simulink model "HybridFEMModel"  (Simulink 7.0)
settings: Solver=FixedStepDiscrete  SolverMode=SingleTasking  StartTime=0.0  StopTime=RunningTime  FixedStep=SampleRate  RelTol=1e-3
values from neighbouring files (symbols this model uses):
  SampleRate = Integrator.Timestep    [HybridFEMSetup_1.m]
undefined symbols (not defined in the file or in its folder): Elements
libraries: simulink x2
(part 1 of 2)
settings Model: Creator=Tommy  LastModifiedBy=Tommy

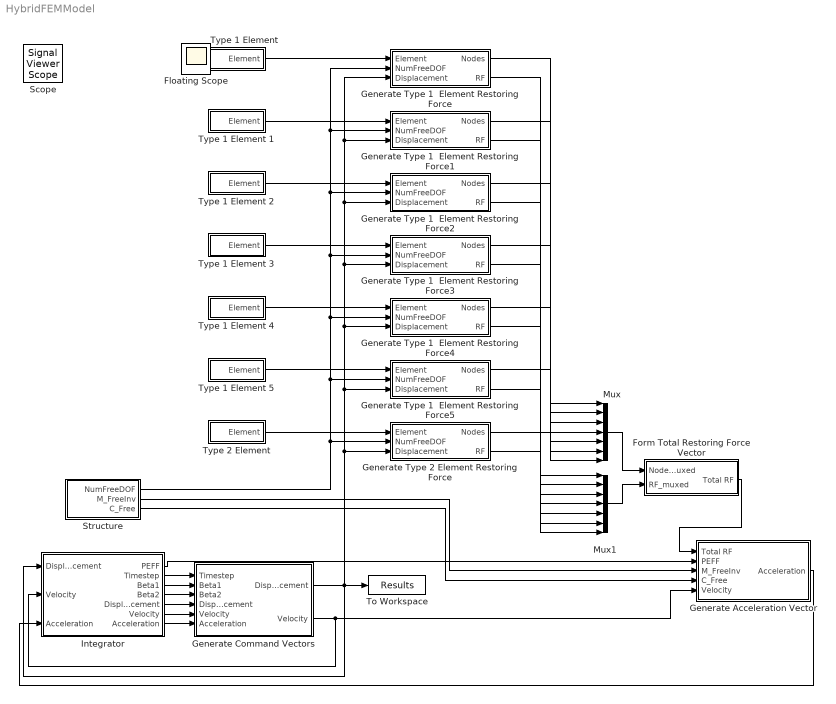
== system HybridFEMModel ==
  Form Total Restoring Force Vector : Subsystem
      mask Type: Form Restoring Force Vector
      mask Description:
      | Takes the restoring force vectors from each Element and combines them to form a total restoring force vector.
      | 
      | Connect the "Nodes_muxed" signal to the output of a Mux block which takes in all the Element "Nodes" outputs in order of ID.
      | 
      | Connect the "RF_muxed" signal to the output of a Mux block which takes in all the Element "RF" outputs in order of ID.
  Generate Acceleration Vector : Subsystem
      mask Type: Generate Acceleration Vector
      mask Description:
      | Takes the total restoring force vector and Integration parameters and generates the next step acceleration vector.
      | 
      | Connect the "Total RF" input to the output of the "Form Total Restoring Force Vector" block.
      | 
      | Connect the "PEFF", "M_Free_Inv" (MassMatrixFreeInv) and "C_Free" (DampingMatrixFree) to the "Structure" block.
      | 
      | Connect the "Velocity" input to the output of the "Generate Command Vectors" block
  Generate Command Vectors : Subsystem
      mask Type: Generate Command Vectors
      mask Description:
      | Generates the Displacement and Velocity vectors using the CR Algorithm.
      | 
      | Connect all inputs to the outputs of the "Integrator" block.
  Generate Type 1  Element Restoring Force : Subsystem
      mask Type: Generate Type 1 Element Restoring Force
      mask Description:
      | Generates the Restoring Force vector for a Type 1 Element
      | 
      | Connect the "Element" input to a "Type 1 Element" block.
      | 
      | Connect the "NumFreeDOF" input to the output of a "Structure" block.
      | 
      | Connect the "Displacement" input to the output of the "Generate Command Vectors" block.
  Generate Type 1  Element Restoring Force1 : Subsystem
      mask Type: Generate Type 1 Element Restoring Force
      mask Description:
      | Generates the Restoring Force vector for a Type 1 Element
      | 
      | Connect the "Element" input to a "Type 1 Element" block.
      | 
      | Connect the "NumFreeDOF" input to the output of a "Structure" block.
      | 
      | Connect the "Displacement" input to the output of the "Generate Command Vectors" block.
  Generate Type 1  Element Restoring Force2 : Subsystem
      mask Type: Generate Type 1 Element Restoring Force
      mask Description:
      | Generates the Restoring Force vector for a Type 1 Element
      | 
      | Connect the "Element" input to a "Type 1 Element" block.
      | 
      | Connect the "NumFreeDOF" input to the output of a "Structure" block.
      | 
      | Connect the "Displacement" input to the output of the "Generate Command Vectors" block.
  Generate Type 1  Element Restoring Force3 : Subsystem
      mask Type: Generate Type 1 Element Restoring Force
      mask Description:
      | Generates the Restoring Force vector for a Type 1 Element
      | 
      | Connect the "Element" input to a "Type 1 Element" block.
      | 
      | Connect the "NumFreeDOF" input to the output of a "Structure" block.
      | 
      | Connect the "Displacement" input to the output of the "Generate Command Vectors" block.
  Generate Type 1  Element Restoring Force4 : Subsystem
      mask Type: Generate Type 1 Element Restoring Force
      mask Description:
      | Generates the Restoring Force vector for a Type 1 Element
      | 
      | Connect the "Element" input to a "Type 1 Element" block.
      | 
      | Connect the "NumFreeDOF" input to the output of a "Structure" block.
      | 
      | Connect the "Displacement" input to the output of the "Generate Command Vectors" block.
  Generate Type 1  Element Restoring Force5 : Subsystem
      mask Type: Generate Type 1 Element Restoring Force
      mask Description:
      | Generates the Restoring Force vector for a Type 1 Element
      | 
      | Connect the "Element" input to a "Type 1 Element" block.
      | 
      | Connect the "NumFreeDOF" input to the output of a "Structure" block.
      | 
      | Connect the "Displacement" input to the output of the "Generate Command Vectors" block.
  Generate Type 2 Element Restoring Force : Subsystem
      mask Type: Generate Type 2 Element Restoring Force
      mask Description:
      | Generates the Restoring Force vector for a Type 2 Element
      | 
      | Connect the "Element" input to a "Type 2 Element" block.
      | 
      | Connect the "NumFreeDOF" input to the output of a "Structure" block.
      | 
      | Connect the "Displacement" input to the output of the "Generate Command Vectors" block.
  Integrator : Subsystem
      mask Type: Integrator
      mask Description:
      | The Integrator structure is pulled from the MATLAB workspace after running the initialization script.
      | 
      | Connect the Displacement and Velocity inputs to the outputs of the "Generate Command Vectors" block.
      | 
      | Connect the Acceleration input to the output of the "Generate Acceleration Vector" block
  Mux : Mux  Inputs=7
  Mux1 : Mux  Inputs=7
  Structure : Subsystem
      mask Type: Structure Data Source
      mask Description: The Structure data is pulled from the MATLAB workspace after running the initialization file
  To Workspace : ToWorkspace  VariableName=Results  SampleTime=SampleRate  SaveFormat=Array
  "Type 1 Element " : Subsystem  mask(Element Type 1){id=1}
      mask prompts: id "Element ID:"
      mask help: Enter the ID for this element corresponding with the input configuration file
  Type 1 Element 1 : Subsystem  mask(Element Type 1){id=2}
      mask prompts: id "Element ID:"
      mask help: Enter the ID for this element corresponding with the input configuration file
  Type 1 Element 2 : Subsystem  mask(Element Type 1){id=3}
      mask prompts: id "Element ID:"
      mask help: Enter the ID for this element corresponding with the input configuration file
  Type 1 Element 3 : Subsystem  mask(Element Type 1){id=4}
      mask prompts: id "Element ID:"
      mask help: Enter the ID for this element corresponding with the input configuration file
  Type 1 Element 4 : Subsystem  mask(Element Type 1){id=5}
      mask prompts: id "Element ID:"
      mask help: Enter the ID for this element corresponding with the input configuration file
  Type 1 Element 5 : Subsystem  mask(Element Type 1){id=6}
      mask prompts: id "Element ID:"
      mask help: Enter the ID for this element corresponding with the input configuration file
  Type 2 Element : Subsystem  mask(Element Type 2){id=7}
      mask prompts: id "Element ID:"
      mask help: Enter the ID for this element corresponding with the input configuration file
  Floating Scope : Scope
      settings: Floating=on
  Scope : SignalViewerScope  IOType=viewer  RefreshTime=0.035000
  wires:
  "Type 1 Element "/1(Element) -> Generate Type 1  Element Restoring Force/1(Element)
  Type 1 Element 1/1(Element) -> Generate Type 1  Element Restoring Force1/1(Element)
  Type 1 Element 2/1(Element) -> Generate Type 1  Element Restoring Force2/1(Element)
  Type 1 Element 3/1(Element) -> Generate Type 1  Element Restoring Force3/1(Element)
  Type 1 Element 4/1(Element) -> Generate Type 1  Element Restoring Force4/1(Element)
  Type 1 Element 5/1(Element) -> Generate Type 1  Element Restoring Force5/1(Element)
  Type 2 Element/1(Element) -> Generate Type 2 Element Restoring Force/1(Element)
  Integrator/5(Displacement) -> Generate Command Vectors/4("Displacement ")
  Structure/1(NumFreeDOF) -> Generate Type 1  Element Restoring Force/2(NumFreeDOF), Generate Type 1  Element Restoring Force1/2(NumFreeDOF), Generate Type 1  Element Restoring Force2/2(NumFreeDOF), Generate Type 1  Element Restoring Force3/2(NumFreeDOF), Generate Type 1  Element Restoring Force4/2(NumFreeDOF), Generate Type 1  Element Restoring Force5/2(NumFreeDOF), Generate Type 2 Element Restoring Force/2(NumFreeDOF)
  Generate Command Vectors/1(Displacement) -> Generate Type 1  Element Restoring Force/3(Displacement), Generate Type 1  Element Restoring Force1/3(Displacement), Generate Type 1  Element Restoring Force2/3(Displacement), Generate Type 1  Element Restoring Force3/3(Displacement), Generate Type 1  Element Restoring Force4/3(Displacement), Generate Type 1  Element Restoring Force5/3(Displacement), Generate Type 2 Element Restoring Force/3(Displacement), Integrator/1("Displacement "), To Workspace/1
  Form Total Restoring Force Vector/1(Total RF) -> Generate Acceleration Vector/1(Total RF)
  Mux/1 -> Form Total Restoring Force Vector/1(Nodes_Muxed)
  Mux1/1 -> Form Total Restoring Force Vector/2(RF_muxed)
  Generate Type 1  Element Restoring Force/1(Nodes) -> Mux/1
  Generate Type 1  Element Restoring Force1/1(Nodes) -> Mux/2
  Generate Type 1  Element Restoring Force2/1(Nodes) -> Mux/3
  Generate Type 1  Element Restoring Force3/1(Nodes) -> Mux/4
  Generate Type 1  Element Restoring Force4/1(Nodes) -> Mux/5
  Generate Type 1  Element Restoring Force5/1(Nodes) -> Mux/6
  Generate Type 2 Element Restoring Force/1(Nodes) -> Mux/7
  Generate Type 1  Element Restoring Force/2(RF) -> Mux1/1
  Generate Type 1  Element Restoring Force1/2(RF) -> Mux1/2
  Generate Type 1  Element Restoring Force2/2(RF) -> Mux1/3
  Generate Type 1  Element Restoring Force3/2(RF) -> Mux1/4
  Generate Type 1  Element Restoring Force4/2(RF) -> Mux1/5
  Generate Type 1  Element Restoring Force5/2(RF) -> Mux1/6
  Generate Type 2 Element Restoring Force/2(RF) -> Mux1/7
  Integrator/1(PEFF) -> Generate Acceleration Vector/2(PEFF)
  Generate Command Vectors/2(Velocity) -> Integrator/2("Velocity "), Generate Acceleration Vector/5(Velocity)
  Structure/2(M_FreeInv) -> Generate Acceleration Vector/3(M_FreeInv)
  Structure/3(C_Free) -> Generate Acceleration Vector/4(C_Free)
  Generate Acceleration Vector/1(Acceleration) -> Integrator/3("Acceleration ")
  Integrator/2(Timestep) -> Generate Command Vectors/1(Timestep)
  Integrator/3(Beta1) -> Generate Command Vectors/2(Beta1)
  Integrator/4(Beta2) -> Generate Command Vectors/3(Beta2)
  Integrator/6(Velocity) -> Generate Command Vectors/5("Velocity ")
  Integrator/7(Acceleration) -> Generate Command Vectors/6(Acceleration)

== system HybridFEMModel/Form Total Restoring Force Vector ==
  Nodes_Muxed : Inport  OutDataType=sfix(16)  OutScaling=2^0
  RF_muxed : Inport  Port=2  OutDataType=sfix(16)  OutScaling=2^0
  Form Restoring Force Vector : Stateflow chart
  Total RF : Outport  OutDataType=sfix(16)  OutScaling=2^0
  wires:
  RF_muxed/1 -> Form Restoring Force Vector/2(RF_muxed)
  Form Restoring Force Vector/1(TotalRF) -> Total RF/1
  Nodes_Muxed/1 -> Form Restoring Force Vector/1(Nodes_muxed)

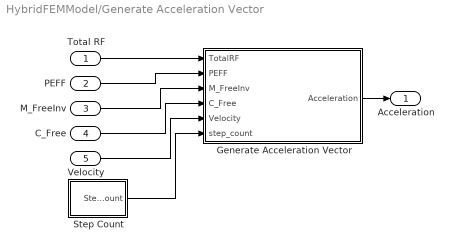
== system HybridFEMModel/Generate Acceleration Vector ==
  Total RF : Inport  OutDataType=sfix(16)  OutScaling=2^0
  PEFF : Inport  Port=2  OutDataType=sfix(16)  OutScaling=2^0
  M_FreeInv : Inport  Port=3  OutDataType=sfix(16)  OutScaling=2^0
  C_Free : Inport  Port=4  OutDataType=sfix(16)  OutScaling=2^0
  Velocity : Inport  Port=5  OutDataType=sfix(16)  OutScaling=2^0
  Generate Acceleration Vector : Stateflow chart
  Step Count : Subsystem
      mask Type: Step count
      mask Description: Generates the step count
  Acceleration : Outport  OutDataType=sfix(16)  OutScaling=2^0
  wires:
  Step Count/1(Step Count) -> Generate Acceleration Vector/6(step_count)
  Total RF/1 -> Generate Acceleration Vector/1(TotalRF)
  Generate Acceleration Vector/1(Acceleration) -> Acceleration/1
  PEFF/1 -> Generate Acceleration Vector/2(PEFF)
  M_FreeInv/1 -> Generate Acceleration Vector/3(M_FreeInv)
  C_Free/1 -> Generate Acceleration Vector/4(C_Free)
  Velocity/1 -> Generate Acceleration Vector/5(Velocity)

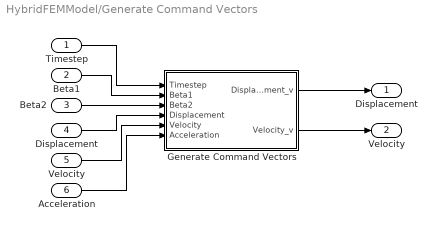
== system HybridFEMModel/Generate Command Vectors ==
  Timestep : Inport  OutDataType=sfix(16)  OutScaling=2^0
  Beta1 : Inport  Port=2  OutDataType=sfix(16)  OutScaling=2^0
  Beta2 : Inport  Port=3  OutDataType=sfix(16)  OutScaling=2^0
  "Displacement " : Inport  Port=4  OutDataType=sfix(16)  OutScaling=2^0
  "Velocity " : Inport  Port=5  OutDataType=sfix(16)  OutScaling=2^0
  Acceleration : Inport  Port=6  OutDataType=sfix(16)  OutScaling=2^0
  Generate Command Vectors : Stateflow chart
  Displacement : Outport  OutDataType=sfix(16)  OutScaling=2^0
  Velocity : Outport  Port=2  OutDataType=sfix(16)  OutScaling=2^0
  wires:
  Generate Command Vectors/1(Displacement_v) -> Displacement/1
  Generate Command Vectors/2(Velocity_v) -> Velocity/1
  Timestep/1 -> Generate Command Vectors/1(Timestep)
  Beta1/1 -> Generate Command Vectors/2(Beta1)
  Beta2/1 -> Generate Command Vectors/3(Beta2)
  "Displacement "/1 -> Generate Command Vectors/4(Displacement)
  "Velocity "/1 -> Generate Command Vectors/5(Velocity)
  Acceleration/1 -> Generate Command Vectors/6(Acceleration)

== system HybridFEMModel/Generate Type 1  Element Restoring Force ==
  Element : Inport  OutDataType=sfix(16)  OutScaling=2^0
  NumFreeDOF : Inport  Port=2  OutDataType=sfix(16)  OutScaling=2^0
  Displacement : Inport  Port=3  OutDataType=sfix(16)  OutScaling=2^0
  Type 1 Element RF : Stateflow chart
  Nodes : Outport  OutDataType=sfix(16)  OutScaling=2^0
  RF : Outport  Port=2  OutDataType=sfix(16)  OutScaling=2^0
  wires:
  Type 1 Element RF/1(Nodes) -> Nodes/1
  Type 1 Element RF/2(RF) -> RF/1
  Element/1 -> Type 1 Element RF/1(Element)
  NumFreeDOF/1 -> Type 1 Element RF/2(NumFreeDOF)
  Displacement/1 -> Type 1 Element RF/3(Displacement)

== system HybridFEMModel/Generate Type 1  Element Restoring Force1 ==
  Element : Inport  OutDataType=sfix(16)  OutScaling=2^0
  NumFreeDOF : Inport  Port=2  OutDataType=sfix(16)  OutScaling=2^0
  Displacement : Inport  Port=3  OutDataType=sfix(16)  OutScaling=2^0
  Type 1 Element RF : Stateflow chart
  Nodes : Outport  OutDataType=sfix(16)  OutScaling=2^0
  RF : Outport  Port=2  OutDataType=sfix(16)  OutScaling=2^0
  wires:
  Displacement/1 -> Type 1 Element RF/3(Displacement)
  NumFreeDOF/1 -> Type 1 Element RF/2(NumFreeDOF)
  Element/1 -> Type 1 Element RF/1(Element)
  Type 1 Element RF/2(RF) -> RF/1
  Type 1 Element RF/1(Nodes) -> Nodes/1

== system HybridFEMModel/Generate Type 1  Element Restoring Force2 ==
  Element : Inport  OutDataType=sfix(16)  OutScaling=2^0
  NumFreeDOF : Inport  Port=2  OutDataType=sfix(16)  OutScaling=2^0
  Displacement : Inport  Port=3  OutDataType=sfix(16)  OutScaling=2^0
  Type 1 Element RF : Stateflow chart
  Nodes : Outport  OutDataType=sfix(16)  OutScaling=2^0
  RF : Outport  Port=2  OutDataType=sfix(16)  OutScaling=2^0
  wires:
  Type 1 Element RF/1(Nodes) -> Nodes/1
  Type 1 Element RF/2(RF) -> RF/1
  Element/1 -> Type 1 Element RF/1(Element)
  NumFreeDOF/1 -> Type 1 Element RF/2(NumFreeDOF)
  Displacement/1 -> Type 1 Element RF/3(Displacement)

== system HybridFEMModel/Generate Type 1  Element Restoring Force3 ==
  Element : Inport  OutDataType=sfix(16)  OutScaling=2^0
  NumFreeDOF : Inport  Port=2  OutDataType=sfix(16)  OutScaling=2^0
  Displacement : Inport  Port=3  OutDataType=sfix(16)  OutScaling=2^0
  Type 1 Element RF : Stateflow chart
  Nodes : Outport  OutDataType=sfix(16)  OutScaling=2^0
  RF : Outport  Port=2  OutDataType=sfix(16)  OutScaling=2^0
  wires:
  Displacement/1 -> Type 1 Element RF/3(Displacement)
  NumFreeDOF/1 -> Type 1 Element RF/2(NumFreeDOF)
  Element/1 -> Type 1 Element RF/1(Element)
  Type 1 Element RF/2(RF) -> RF/1
  Type 1 Element RF/1(Nodes) -> Nodes/1

== system HybridFEMModel/Generate Type 1  Element Restoring Force4 ==
  Element : Inport  OutDataType=sfix(16)  OutScaling=2^0
  NumFreeDOF : Inport  Port=2  OutDataType=sfix(16)  OutScaling=2^0
  Displacement : Inport  Port=3  OutDataType=sfix(16)  OutScaling=2^0
  Type 1 Element RF : Stateflow chart
  Nodes : Outport  OutDataType=sfix(16)  OutScaling=2^0
  RF : Outport  Port=2  OutDataType=sfix(16)  OutScaling=2^0
  wires:
  Type 1 Element RF/1(Nodes) -> Nodes/1
  Type 1 Element RF/2(RF) -> RF/1
  Element/1 -> Type 1 Element RF/1(Element)
  NumFreeDOF/1 -> Type 1 Element RF/2(NumFreeDOF)
  Displacement/1 -> Type 1 Element RF/3(Displacement)

== system HybridFEMModel/Generate Type 1  Element Restoring Force5 ==
  Element : Inport  OutDataType=sfix(16)  OutScaling=2^0
  NumFreeDOF : Inport  Port=2  OutDataType=sfix(16)  OutScaling=2^0
  Displacement : Inport  Port=3  OutDataType=sfix(16)  OutScaling=2^0
  Type 1 Element RF : Stateflow chart
  Nodes : Outport  OutDataType=sfix(16)  OutScaling=2^0
  RF : Outport  Port=2  OutDataType=sfix(16)  OutScaling=2^0
  wires:
  Displacement/1 -> Type 1 Element RF/3(Displacement)
  NumFreeDOF/1 -> Type 1 Element RF/2(NumFreeDOF)
  Element/1 -> Type 1 Element RF/1(Element)
  Type 1 Element RF/2(RF) -> RF/1
  Type 1 Element RF/1(Nodes) -> Nodes/1

== system HybridFEMModel/Generate Type 2 Element Restoring Force ==
  Element : Inport  OutDataType=sfix(16)  OutScaling=2^0
  NumFreeDOF : Inport  Port=2  OutDataType=sfix(16)  OutScaling=2^0
  Displacement : Inport  Port=3  OutDataType=sfix(16)  OutScaling=2^0
  Type 2 Element RF : Stateflow chart
  Nodes : Outport  OutDataType=sfix(16)  OutScaling=2^0
  RF : Outport  Port=2  OutDataType=sfix(16)  OutScaling=2^0
  wires:
  Displacement/1 -> Type 2 Element RF/3(Displacement)
  NumFreeDOF/1 -> Type 2 Element RF/2(NumFreeDOF)
  Element/1 -> Type 2 Element RF/1(Element)
  Type 2 Element RF/2(RF) -> RF/1
  Type 2 Element RF/1(Nodes) -> Nodes/1

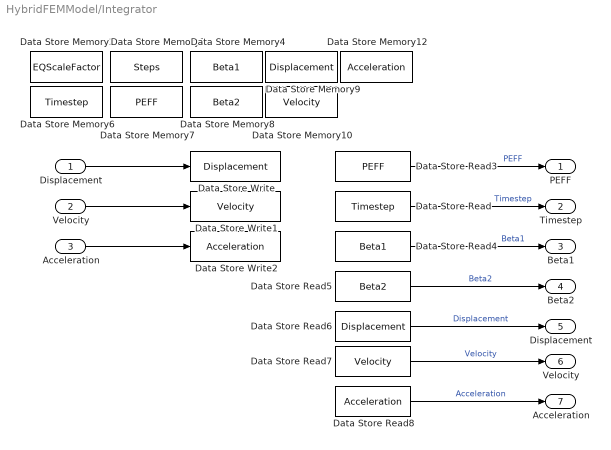
== system HybridFEMModel/Integrator ==
  "Displacement " : Inport  OutDataType=sfix(16)  OutScaling=2^0
  "Velocity " : Inport  Port=2  OutDataType=sfix(16)  OutScaling=2^0
  "Acceleration " : Inport  Port=3  OutDataType=sfix(16)  OutScaling=2^0
  Data Store Memory10 : DataStoreMemory  DataStoreName=Velocity  InitialValue=Integrator.Velocity  OutDataType=sfix(16)  OutScaling=2^0
  Data Store Memory12 : DataStoreMemory  DataStoreName=Acceleration  InitialValue=Integrator.Acceleration  OutDataType=sfix(16)  OutScaling=2^0
  Data Store Memory2 : DataStoreMemory  DataStoreName=EQScaleFactor  InitialValue=Integrator.EQScaleFactor  OutDataType=sfix(16)  OutScaling=2^0
  Data Store Memory3 : DataStoreMemory  DataStoreName=Steps  InitialValue=Integrator.Steps  OutDataType=sfix(16)  OutScaling=2^0
  Data Store Memory4 : DataStoreMemory  DataStoreName=Beta1  InitialValue=Integrator.Beta1  OutDataType=sfix(16)  OutScaling=2^0
  Data Store Memory6 : DataStoreMemory  DataStoreName=Timestep  InitialValue=Integrator.Timestep  OutDataType=sfix(16)  OutScaling=2^0
  Data Store Memory7 : DataStoreMemory  DataStoreName=PEFF  InitialValue=Integrator.PEFF  OutDataType=sfix(16)  OutScaling=2^0
  Data Store Memory8 : DataStoreMemory  DataStoreName=Beta2  InitialValue=Integrator.Beta2  OutDataType=sfix(16)  OutScaling=2^0
  Data Store Memory9 : DataStoreMemory  DataStoreName=Displacement  InitialValue=Integrator.Displacement  OutDataType=sfix(16)  OutScaling=2^0
  Data Store Read : DataStoreRead  DataStoreName=Timestep  SampleTime=SampleRate
  Data Store Read3 : DataStoreRead  DataStoreName=PEFF  SampleTime=SampleRate
  Data Store Read4 : DataStoreRead  DataStoreName=Beta1  SampleTime=SampleRate
  Data Store Read5 : DataStoreRead  DataStoreName=Beta2  SampleTime=SampleRate
  Data Store Read6 : DataStoreRead  DataStoreName=Displacement  SampleTime=SampleRate
  Data Store Read7 : DataStoreRead  DataStoreName=Velocity  SampleTime=SampleRate
  Data Store Read8 : DataStoreRead  DataStoreName=Acceleration  SampleTime=SampleRate
  Data Store Write : DataStoreWrite  DataStoreName=Displacement  SampleTime=SampleRate
  Data Store Write1 : DataStoreWrite  DataStoreName=Velocity  SampleTime=SampleRate
  Data Store Write2 : DataStoreWrite  DataStoreName=Acceleration  SampleTime=SampleRate
  PEFF : Outport  OutDataType=sfix(16)  OutScaling=2^0
  Timestep : Outport  Port=2  OutDataType=sfix(16)  OutScaling=2^0
  Beta1 : Outport  Port=3  OutDataType=sfix(16)  OutScaling=2^0
  Beta2 : Outport  Port=4  OutDataType=sfix(16)  OutScaling=2^0
  Displacement : Outport  Port=5  OutDataType=sfix(16)  OutScaling=2^0
  Velocity : Outport  Port=6  OutDataType=sfix(16)  OutScaling=2^0
  Acceleration : Outport  Port=7  OutDataType=sfix(16)  OutScaling=2^0
  wires:
  Data Store Read/1 -> Timestep/1  "Timestep"
  "Acceleration "/1 -> Data Store Write2/1
  "Velocity "/1 -> Data Store Write1/1
  "Displacement "/1 -> Data Store Write/1
  Data Store Read3/1 -> PEFF/1  "PEFF"
  Data Store Read4/1 -> Beta1/1  "Beta1"
  Data Store Read5/1 -> Beta2/1  "Beta2"
  Data Store Read6/1 -> Displacement/1  "Displacement"
  Data Store Read7/1 -> Velocity/1  "Velocity"
  Data Store Read8/1 -> Acceleration/1  "Acceleration"

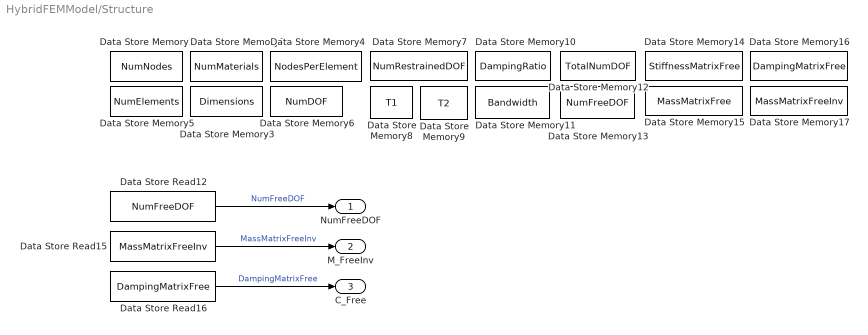
== system HybridFEMModel/Structure ==
  Data Store Memory1 : DataStoreMemory  DataStoreName=NumNodes  InitialValue=Structure.NumNodes  OutDataType=sfix(16)  OutScaling=2^0
  Data Store Memory10 : DataStoreMemory  DataStoreName=DampingRatio  InitialValue=Structure.DampingRatio  OutDataType=sfix(16)  OutScaling=2^0
  Data Store Memory11 : DataStoreMemory  DataStoreName=Bandwidth  InitialValue=Structure.Bandwidth  OutDataType=sfix(16)  OutScaling=2^0
  Data Store Memory12 : DataStoreMemory  DataStoreName=TotalNumDOF  InitialValue=Structure.TotalNumDOF  OutDataType=sfix(16)  OutScaling=2^0
  Data Store Memory13 : DataStoreMemory  DataStoreName=NumFreeDOF  InitialValue=Structure.NumFreeDOF  OutDataType=sfix(16)  OutScaling=2^0
  Data Store Memory14 : DataStoreMemory  DataStoreName=StiffnessMatrixFree  InitialValue=Structure.StiffnessMatrixFree  OutDataType=sfix(16)  OutScaling=2^0
  Data Store Memory15 : DataStoreMemory  DataStoreName=MassMatrixFree  InitialValue=Structure.MassMatrixFree  OutDataType=sfix(16)  OutScaling=2^0
  Data Store Memory16 : DataStoreMemory  DataStoreName=DampingMatrixFree  InitialValue=Structure.DampingMatrixFree  OutDataType=sfix(16)  OutScaling=2^0
  Data Store Memory17 : DataStoreMemory  DataStoreName=MassMatrixFreeInv  InitialValue=Structure.MassMatrixFreeInv  OutDataType=sfix(16)  OutScaling=2^0
  Data Store Memory2 : DataStoreMemory  DataStoreName=NumMaterials  InitialValue=Structure.NumMaterials  OutDataType=sfix(16)  OutScaling=2^0
  Data Store Memory3 : DataStoreMemory  DataStoreName=Dimensions  InitialValue=Structure.Dimensions  OutDataType=sfix(16)  OutScaling=2^0
  Data Store Memory4 : DataStoreMemory  DataStoreName=NodesPerElement  InitialValue=Structure.NodesPerElement  OutDataType=sfix(16)  OutScaling=2^0
  Data Store Memory5 : DataStoreMemory  DataStoreName=NumElements  InitialValue=Structure.NumElements  OutDataType=sfix(16)  OutScaling=2^0
  Data Store Memory6 : DataStoreMemory  DataStoreName=NumDOF  InitialValue=Structure.NumDOF  OutDataType=sfix(16)  OutScaling=2^0
  Data Store Memory7 : DataStoreMemory  DataStoreName=NumRestrainedDOF  InitialValue=Structure.NumRestrainedDOF  OutDataType=sfix(16)  OutScaling=2^0
  Data Store Memory8 : DataStoreMemory  DataStoreName=T1  InitialValue=Structure.T1  OutDataType=sfix(16)  OutScaling=2^0
  Data Store Memory9 : DataStoreMemory  DataStoreName=T2  InitialValue=Structure.T2  OutDataType=sfix(16)  OutScaling=2^0
  Data Store Read12 : DataStoreRead  DataStoreName=NumFreeDOF  SampleTime=SampleRate
  Data Store Read15 : DataStoreRead  DataStoreName=MassMatrixFreeInv  SampleTime=SampleRate
  Data Store Read16 : DataStoreRead  DataStoreName=DampingMatrixFree  SampleTime=SampleRate
  NumFreeDOF : Outport  OutDataType=sfix(16)  OutScaling=2^0
  M_FreeInv : Outport  Port=2  OutDataType=sfix(16)  OutScaling=2^0
  C_Free : Outport  Port=3  OutDataType=sfix(16)  OutScaling=2^0
  wires:
  Data Store Read12/1 -> NumFreeDOF/1  "NumFreeDOF"
  Data Store Read15/1 -> M_FreeInv/1  "MassMatrixFreeInv"
  Data Store Read16/1 -> C_Free/1  "DampingMatrixFree"

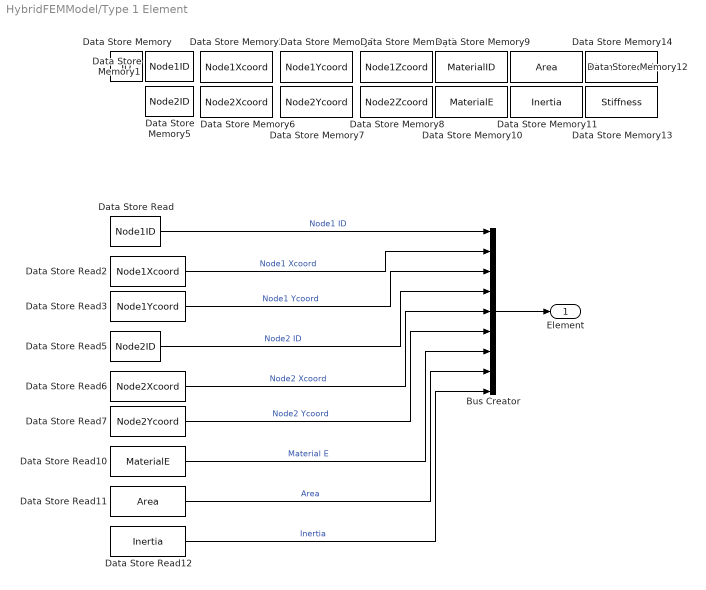
== system HybridFEMModel/Type 1 Element  ==
  Bus Creator : BusCreator  Inputs=9
  Data Store Memory : DataStoreMemory  DataStoreName=ID  InitialValue=Elements(id).ID  OutDataType=sfix(16)  OutScaling=2^0
  Data Store Memory1 : DataStoreMemory  DataStoreName=Node1ID  InitialValue=Elements(id).Nodes(1).ID  OutDataType=sfix(16)  OutScaling=2^0
  Data Store Memory10 : DataStoreMemory  DataStoreName=MaterialE  InitialValue=Elements(id).Material(1).E  OutDataType=sfix(16)  OutScaling=2^0
  Data Store Memory11 : DataStoreMemory  DataStoreName=Inertia  InitialValue=Elements(id).Inertia  OutDataType=sfix(16)  OutScaling=2^0
  Data Store Memory12 : DataStoreMemory  DataStoreName=Area  InitialValue=Elements(id).Area  OutDataType=sfix(16)  OutScaling=2^0
  Data Store Memory13 : DataStoreMemory  DataStoreName=Stiffness  InitialValue=Elements(id).Stiffness  OutDataType=sfix(16)  OutScaling=2^0
  Data Store Memory14 : DataStoreMemory  DataStoreName=ElemDistLoad  InitialValue=Elements(id).ElemDistLoad  OutDataType=sfix(16)  OutScaling=2^0
  Data Store Memory2 : DataStoreMemory  DataStoreName=Node1Xcoord  InitialValue=Elements(id).Nodes(1).Xcoord  OutDataType=sfix(16)  OutScaling=2^0
  Data Store Memory3 : DataStoreMemory  DataStoreName=Node1Ycoord  InitialValue=Elements(id).Nodes(1).Ycoord  OutDataType=sfix(16)  OutScaling=2^0
  Data Store Memory4 : DataStoreMemory  DataStoreName=Node1Zcoord  InitialValue=Elements(id).Nodes(1).Zcoord  OutDataType=sfix(16)  OutScaling=2^0
  Data Store Memory5 : DataStoreMemory  DataStoreName=Node2ID  InitialValue=Elements(id).Nodes(2).ID  OutDataType=sfix(16)  OutScaling=2^0
  Data Store Memory6 : DataStoreMemory  DataStoreName=Node2Xcoord  InitialValue=Elements(id).Nodes(2).Xcoord  OutDataType=sfix(16)  OutScaling=2^0
  Data Store Memory7 : DataStoreMemory  DataStoreName=Node2Ycoord  InitialValue=Elements(id).Nodes(2).Ycoord  OutDataType=sfix(16)  OutScaling=2^0
  Data Store Memory8 : DataStoreMemory  DataStoreName=Node2Zcoord  InitialValue=Elements(id).Nodes(2).Zcoord  OutDataType=sfix(16)  OutScaling=2^0
  Data Store Memory9 : DataStoreMemory  DataStoreName=MaterialID  InitialValue=Elements(id).Material(1).ID  OutDataType=sfix(16)  OutScaling=2^0
  Data Store Read : DataStoreRead  DataStoreName=Node1ID  SampleTime=SampleRate
  Data Store Read10 : DataStoreRead  DataStoreName=MaterialE  SampleTime=SampleRate
  Data Store Read11 : DataStoreRead  DataStoreName=Area  SampleTime=SampleRate
  Data Store Read12 : DataStoreRead  DataStoreName=Inertia  SampleTime=SampleRate
  Data Store Read2 : DataStoreRead  DataStoreName=Node1Xcoord  SampleTime=SampleRate
  Data Store Read3 : DataStoreRead  DataStoreName=Node1Ycoord  SampleTime=SampleRate
  Data Store Read5 : DataStoreRead  DataStoreName=Node2ID  SampleTime=SampleRate
  Data Store Read6 : DataStoreRead  DataStoreName=Node2Xcoord  SampleTime=SampleRate
  Data Store Read7 : DataStoreRead  DataStoreName=Node2Ycoord  SampleTime=SampleRate
  Element : Outport  OutDataType=sfix(16)  OutScaling=2^0
  wires:
  Bus Creator/1 -> Element/1
  Data Store Read/1 -> Bus Creator/1  "Node1 ID"
  Data Store Read2/1 -> Bus Creator/2  "Node1 Xcoord"
  Data Store Read3/1 -> Bus Creator/3  "Node1 Ycoord"
  Data Store Read5/1 -> Bus Creator/4  "Node2 ID"
  Data Store Read6/1 -> Bus Creator/5  "Node2 Xcoord"
  Data Store Read7/1 -> Bus Creator/6  "Node2 Ycoord"
  Data Store Read10/1 -> Bus Creator/7  "Material E"
  Data Store Read11/1 -> Bus Creator/8  "Area"
  Data Store Read12/1 -> Bus Creator/9  "Inertia"

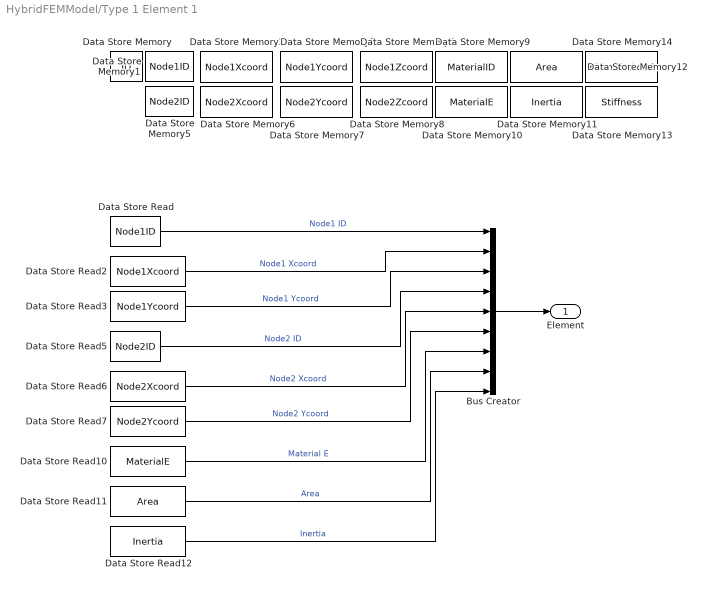
== system HybridFEMModel/Type 1 Element 1 ==
  Bus Creator : BusCreator  Inputs=9
  Data Store Memory : DataStoreMemory  DataStoreName=ID  InitialValue=Elements(id).ID  OutDataType=sfix(16)  OutScaling=2^0
  Data Store Memory1 : DataStoreMemory  DataStoreName=Node1ID  InitialValue=Elements(id).Nodes(1).ID  OutDataType=sfix(16)  OutScaling=2^0
  Data Store Memory10 : DataStoreMemory  DataStoreName=MaterialE  InitialValue=Elements(id).Material(1).E  OutDataType=sfix(16)  OutScaling=2^0
  Data Store Memory11 : DataStoreMemory  DataStoreName=Inertia  InitialValue=Elements(id).Inertia  OutDataType=sfix(16)  OutScaling=2^0
  Data Store Memory12 : DataStoreMemory  DataStoreName=Area  InitialValue=Elements(id).Area  OutDataType=sfix(16)  OutScaling=2^0
  Data Store Memory13 : DataStoreMemory  DataStoreName=Stiffness  InitialValue=Elements(id).Stiffness  OutDataType=sfix(16)  OutScaling=2^0
  Data Store Memory14 : DataStoreMemory  DataStoreName=ElemDistLoad  InitialValue=Elements(id).ElemDistLoad  OutDataType=sfix(16)  OutScaling=2^0
  Data Store Memory2 : DataStoreMemory  DataStoreName=Node1Xcoord  InitialValue=Elements(id).Nodes(1).Xcoord  OutDataType=sfix(16)  OutScaling=2^0
  Data Store Memory3 : DataStoreMemory  DataStoreName=Node1Ycoord  InitialValue=Elements(id).Nodes(1).Ycoord  OutDataType=sfix(16)  OutScaling=2^0
  Data Store Memory4 : DataStoreMemory  DataStoreName=Node1Zcoord  InitialValue=Elements(id).Nodes(1).Zcoord  OutDataType=sfix(16)  OutScaling=2^0
  Data Store Memory5 : DataStoreMemory  DataStoreName=Node2ID  InitialValue=Elements(id).Nodes(2).ID  OutDataType=sfix(16)  OutScaling=2^0
  Data Store Memory6 : DataStoreMemory  DataStoreName=Node2Xcoord  InitialValue=Elements(id).Nodes(2).Xcoord  OutDataType=sfix(16)  OutScaling=2^0
  Data Store Memory7 : DataStoreMemory  DataStoreName=Node2Ycoord  InitialValue=Elements(id).Nodes(2).Ycoord  OutDataType=sfix(16)  OutScaling=2^0
  Data Store Memory8 : DataStoreMemory  DataStoreName=Node2Zcoord  InitialValue=Elements(id).Nodes(2).Zcoord  OutDataType=sfix(16)  OutScaling=2^0
  Data Store Memory9 : DataStoreMemory  DataStoreName=MaterialID  InitialValue=Elements(id).Material(1).ID  OutDataType=sfix(16)  OutScaling=2^0
  Data Store Read : DataStoreRead  DataStoreName=Node1ID  SampleTime=SampleRate
  Data Store Read10 : DataStoreRead  DataStoreName=MaterialE  SampleTime=SampleRate
  Data Store Read11 : DataStoreRead  DataStoreName=Area  SampleTime=SampleRate
  Data Store Read12 : DataStoreRead  DataStoreName=Inertia  SampleTime=SampleRate
  Data Store Read2 : DataStoreRead  DataStoreName=Node1Xcoord  SampleTime=SampleRate
  Data Store Read3 : DataStoreRead  DataStoreName=Node1Ycoord  SampleTime=SampleRate
  Data Store Read5 : DataStoreRead  DataStoreName=Node2ID  SampleTime=SampleRate
  Data Store Read6 : DataStoreRead  DataStoreName=Node2Xcoord  SampleTime=SampleRate
  Data Store Read7 : DataStoreRead  DataStoreName=Node2Ycoord  SampleTime=SampleRate
  Element : Outport  OutDataType=sfix(16)  OutScaling=2^0
  wires:
  Data Store Read12/1 -> Bus Creator/9  "Inertia"
  Data Store Read11/1 -> Bus Creator/8  "Area"
  Data Store Read10/1 -> Bus Creator/7  "Material E"
  Data Store Read7/1 -> Bus Creator/6  "Node2 Ycoord"
  Data Store Read6/1 -> Bus Creator/5  "Node2 Xcoord"
  Data Store Read5/1 -> Bus Creator/4  "Node2 ID"
  Data Store Read3/1 -> Bus Creator/3  "Node1 Ycoord"
  Data Store Read2/1 -> Bus Creator/2  "Node1 Xcoord"
  Data Store Read/1 -> Bus Creator/1  "Node1 ID"
  Bus Creator/1 -> Element/1

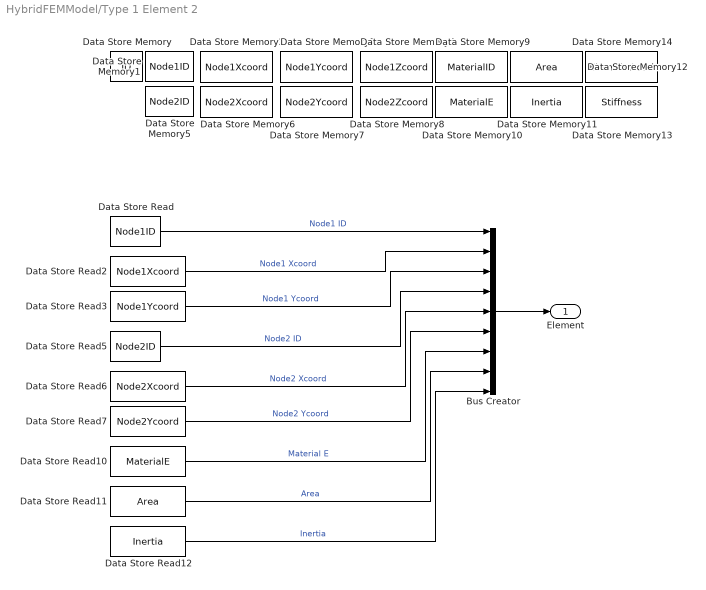
== system HybridFEMModel/Type 1 Element 2 ==
  Bus Creator : BusCreator  Inputs=9
  Data Store Memory : DataStoreMemory  DataStoreName=ID  InitialValue=Elements(id).ID  OutDataType=sfix(16)  OutScaling=2^0
  Data Store Memory1 : DataStoreMemory  DataStoreName=Node1ID  InitialValue=Elements(id).Nodes(1).ID  OutDataType=sfix(16)  OutScaling=2^0
  Data Store Memory10 : DataStoreMemory  DataStoreName=MaterialE  InitialValue=Elements(id).Material(1).E  OutDataType=sfix(16)  OutScaling=2^0
  Data Store Memory11 : DataStoreMemory  DataStoreName=Inertia  InitialValue=Elements(id).Inertia  OutDataType=sfix(16)  OutScaling=2^0
  Data Store Memory12 : DataStoreMemory  DataStoreName=Area  InitialValue=Elements(id).Area  OutDataType=sfix(16)  OutScaling=2^0
  Data Store Memory13 : DataStoreMemory  DataStoreName=Stiffness  InitialValue=Elements(id).Stiffness  OutDataType=sfix(16)  OutScaling=2^0
  Data Store Memory14 : DataStoreMemory  DataStoreName=ElemDistLoad  InitialValue=Elements(id).ElemDistLoad  OutDataType=sfix(16)  OutScaling=2^0
  Data Store Memory2 : DataStoreMemory  DataStoreName=Node1Xcoord  InitialValue=Elements(id).Nodes(1).Xcoord  OutDataType=sfix(16)  OutScaling=2^0
  Data Store Memory3 : DataStoreMemory  DataStoreName=Node1Ycoord  InitialValue=Elements(id).Nodes(1).Ycoord  OutDataType=sfix(16)  OutScaling=2^0
  Data Store Memory4 : DataStoreMemory  DataStoreName=Node1Zcoord  InitialValue=Elements(id).Nodes(1).Zcoord  OutDataType=sfix(16)  OutScaling=2^0
  Data Store Memory5 : DataStoreMemory  DataStoreName=Node2ID  InitialValue=Elements(id).Nodes(2).ID  OutDataType=sfix(16)  OutScaling=2^0
  Data Store Memory6 : DataStoreMemory  DataStoreName=Node2Xcoord  InitialValue=Elements(id).Nodes(2).Xcoord  OutDataType=sfix(16)  OutScaling=2^0
  Data Store Memory7 : DataStoreMemory  DataStoreName=Node2Ycoord  InitialValue=Elements(id).Nodes(2).Ycoord  OutDataType=sfix(16)  OutScaling=2^0
  Data Store Memory8 : DataStoreMemory  DataStoreName=Node2Zcoord  InitialValue=Elements(id).Nodes(2).Zcoord  OutDataType=sfix(16)  OutScaling=2^0
  Data Store Memory9 : DataStoreMemory  DataStoreName=MaterialID  InitialValue=Elements(id).Material(1).ID  OutDataType=sfix(16)  OutScaling=2^0
  Data Store Read : DataStoreRead  DataStoreName=Node1ID  SampleTime=SampleRate
  Data Store Read10 : DataStoreRead  DataStoreName=MaterialE  SampleTime=SampleRate
  Data Store Read11 : DataStoreRead  DataStoreName=Area  SampleTime=SampleRate
  Data Store Read12 : DataStoreRead  DataStoreName=Inertia  SampleTime=SampleRate
  Data Store Read2 : DataStoreRead  DataStoreName=Node1Xcoord  SampleTime=SampleRate
  Data Store Read3 : DataStoreRead  DataStoreName=Node1Ycoord  SampleTime=SampleRate
  Data Store Read5 : DataStoreRead  DataStoreName=Node2ID  SampleTime=SampleRate
  Data Store Read6 : DataStoreRead  DataStoreName=Node2Xcoord  SampleTime=SampleRate
  Data Store Read7 : DataStoreRead  DataStoreName=Node2Ycoord  SampleTime=SampleRate
  Element : Outport  OutDataType=sfix(16)  OutScaling=2^0
  wires:
  Bus Creator/1 -> Element/1
  Data Store Read/1 -> Bus Creator/1  "Node1 ID"
  Data Store Read2/1 -> Bus Creator/2  "Node1 Xcoord"
  Data Store Read3/1 -> Bus Creator/3  "Node1 Ycoord"
  Data Store Read5/1 -> Bus Creator/4  "Node2 ID"
  Data Store Read6/1 -> Bus Creator/5  "Node2 Xcoord"
  Data Store Read7/1 -> Bus Creator/6  "Node2 Ycoord"
  Data Store Read10/1 -> Bus Creator/7  "Material E"
  Data Store Read11/1 -> Bus Creator/8  "Area"
  Data Store Read12/1 -> Bus Creator/9  "Inertia"

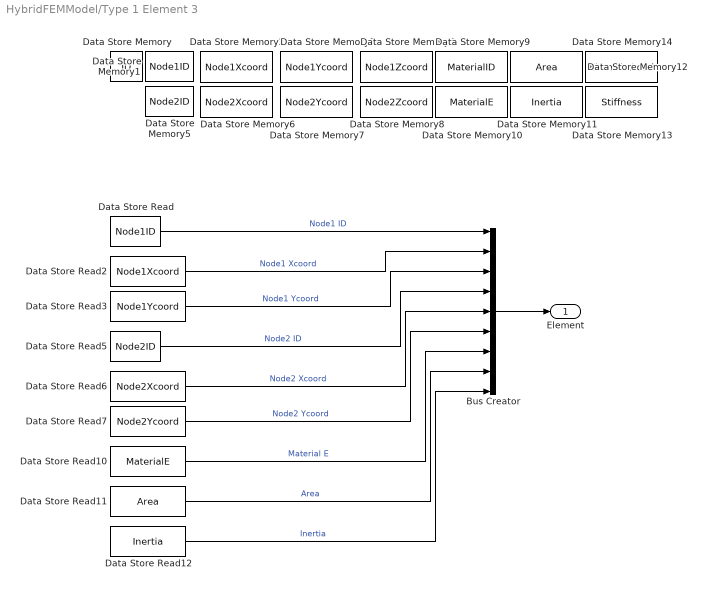
== system HybridFEMModel/Type 1 Element 3 ==
  Bus Creator : BusCreator  Inputs=9
  Data Store Memory : DataStoreMemory  DataStoreName=ID  InitialValue=Elements(id).ID  OutDataType=sfix(16)  OutScaling=2^0
  Data Store Memory1 : DataStoreMemory  DataStoreName=Node1ID  InitialValue=Elements(id).Nodes(1).ID  OutDataType=sfix(16)  OutScaling=2^0
  Data Store Memory10 : DataStoreMemory  DataStoreName=MaterialE  InitialValue=Elements(id).Material(1).E  OutDataType=sfix(16)  OutScaling=2^0
  Data Store Memory11 : DataStoreMemory  DataStoreName=Inertia  InitialValue=Elements(id).Inertia  OutDataType=sfix(16)  OutScaling=2^0
  Data Store Memory12 : DataStoreMemory  DataStoreName=Area  InitialValue=Elements(id).Area  OutDataType=sfix(16)  OutScaling=2^0
  Data Store Memory13 : DataStoreMemory  DataStoreName=Stiffness  InitialValue=Elements(id).Stiffness  OutDataType=sfix(16)  OutScaling=2^0
  Data Store Memory14 : DataStoreMemory  DataStoreName=ElemDistLoad  InitialValue=Elements(id).ElemDistLoad  OutDataType=sfix(16)  OutScaling=2^0
  Data Store Memory2 : DataStoreMemory  DataStoreName=Node1Xcoord  InitialValue=Elements(id).Nodes(1).Xcoord  OutDataType=sfix(16)  OutScaling=2^0
  Data Store Memory3 : DataStoreMemory  DataStoreName=Node1Ycoord  InitialValue=Elements(id).Nodes(1).Ycoord  OutDataType=sfix(16)  OutScaling=2^0
  Data Store Memory4 : DataStoreMemory  DataStoreName=Node1Zcoord  InitialValue=Elements(id).Nodes(1).Zcoord  OutDataType=sfix(16)  OutScaling=2^0
  Data Store Memory5 : DataStoreMemory  DataStoreName=Node2ID  InitialValue=Elements(id).Nodes(2).ID  OutDataType=sfix(16)  OutScaling=2^0
  Data Store Memory6 : DataStoreMemory  DataStoreName=Node2Xcoord  InitialValue=Elements(id).Nodes(2).Xcoord  OutDataType=sfix(16)  OutScaling=2^0
  Data Store Memory7 : DataStoreMemory  DataStoreName=Node2Ycoord  InitialValue=Elements(id).Nodes(2).Ycoord  OutDataType=sfix(16)  OutScaling=2^0
  Data Store Memory8 : DataStoreMemory  DataStoreName=Node2Zcoord  InitialValue=Elements(id).Nodes(2).Zcoord  OutDataType=sfix(16)  OutScaling=2^0
  Data Store Memory9 : DataStoreMemory  DataStoreName=MaterialID  InitialValue=Elements(id).Material(1).ID  OutDataType=sfix(16)  OutScaling=2^0
  Data Store Read : DataStoreRead  DataStoreName=Node1ID  SampleTime=SampleRate
  Data Store Read10 : DataStoreRead  DataStoreName=MaterialE  SampleTime=SampleRate
  Data Store Read11 : DataStoreRead  DataStoreName=Area  SampleTime=SampleRate
  Data Store Read12 : DataStoreRead  DataStoreName=Inertia  SampleTime=SampleRate
  Data Store Read2 : DataStoreRead  DataStoreName=Node1Xcoord  SampleTime=SampleRate
  Data Store Read3 : DataStoreRead  DataStoreName=Node1Ycoord  SampleTime=SampleRate
  Data Store Read5 : DataStoreRead  DataStoreName=Node2ID  SampleTime=SampleRate
  Data Store Read6 : DataStoreRead  DataStoreName=Node2Xcoord  SampleTime=SampleRate
  Data Store Read7 : DataStoreRead  DataStoreName=Node2Ycoord  SampleTime=SampleRate
  Element : Outport  OutDataType=sfix(16)  OutScaling=2^0
  wires:
  Data Store Read12/1 -> Bus Creator/9  "Inertia"
  Data Store Read11/1 -> Bus Creator/8  "Area"
  Data Store Read10/1 -> Bus Creator/7  "Material E"
  Data Store Read7/1 -> Bus Creator/6  "Node2 Ycoord"
  Data Store Read6/1 -> Bus Creator/5  "Node2 Xcoord"
  Data Store Read5/1 -> Bus Creator/4  "Node2 ID"
  Data Store Read3/1 -> Bus Creator/3  "Node1 Ycoord"
  Data Store Read2/1 -> Bus Creator/2  "Node1 Xcoord"
  Data Store Read/1 -> Bus Creator/1  "Node1 ID"
  Bus Creator/1 -> Element/1

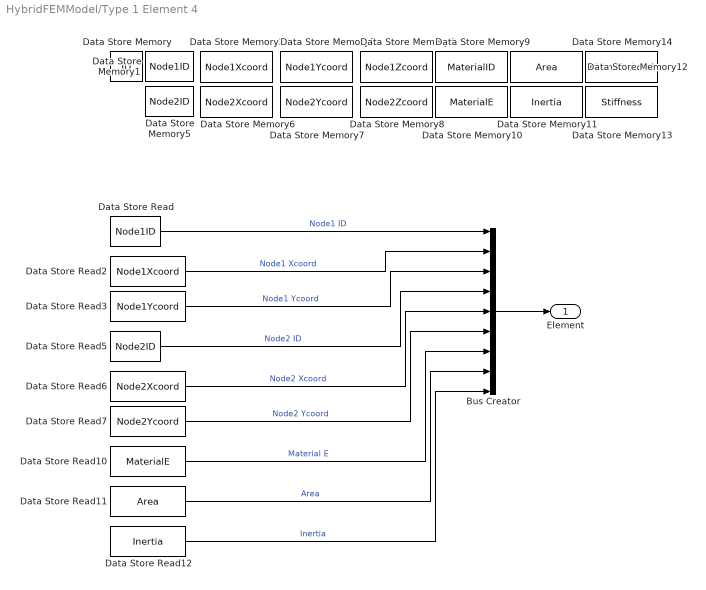
== system HybridFEMModel/Type 1 Element 4 ==
  Bus Creator : BusCreator  Inputs=9
  Data Store Memory : DataStoreMemory  DataStoreName=ID  InitialValue=Elements(id).ID  OutDataType=sfix(16)  OutScaling=2^0
  Data Store Memory1 : DataStoreMemory  DataStoreName=Node1ID  InitialValue=Elements(id).Nodes(1).ID  OutDataType=sfix(16)  OutScaling=2^0
  Data Store Memory10 : DataStoreMemory  DataStoreName=MaterialE  InitialValue=Elements(id).Material(1).E  OutDataType=sfix(16)  OutScaling=2^0
  Data Store Memory11 : DataStoreMemory  DataStoreName=Inertia  InitialValue=Elements(id).Inertia  OutDataType=sfix(16)  OutScaling=2^0
  Data Store Memory12 : DataStoreMemory  DataStoreName=Area  InitialValue=Elements(id).Area  OutDataType=sfix(16)  OutScaling=2^0
  Data Store Memory13 : DataStoreMemory  DataStoreName=Stiffness  InitialValue=Elements(id).Stiffness  OutDataType=sfix(16)  OutScaling=2^0
  Data Store Memory14 : DataStoreMemory  DataStoreName=ElemDistLoad  InitialValue=Elements(id).ElemDistLoad  OutDataType=sfix(16)  OutScaling=2^0
  Data Store Memory2 : DataStoreMemory  DataStoreName=Node1Xcoord  InitialValue=Elements(id).Nodes(1).Xcoord  OutDataType=sfix(16)  OutScaling=2^0
  Data Store Memory3 : DataStoreMemory  DataStoreName=Node1Ycoord  InitialValue=Elements(id).Nodes(1).Ycoord  OutDataType=sfix(16)  OutScaling=2^0
  Data Store Memory4 : DataStoreMemory  DataStoreName=Node1Zcoord  InitialValue=Elements(id).Nodes(1).Zcoord  OutDataType=sfix(16)  OutScaling=2^0
  Data Store Memory5 : DataStoreMemory  DataStoreName=Node2ID  InitialValue=Elements(id).Nodes(2).ID  OutDataType=sfix(16)  OutScaling=2^0
  Data Store Memory6 : DataStoreMemory  DataStoreName=Node2Xcoord  InitialValue=Elements(id).Nodes(2).Xcoord  OutDataType=sfix(16)  OutScaling=2^0
  Data Store Memory7 : DataStoreMemory  DataStoreName=Node2Ycoord  InitialValue=Elements(id).Nodes(2).Ycoord  OutDataType=sfix(16)  OutScaling=2^0
  Data Store Memory8 : DataStoreMemory  DataStoreName=Node2Zcoord  InitialValue=Elements(id).Nodes(2).Zcoord  OutDataType=sfix(16)  OutScaling=2^0
  Data Store Memory9 : DataStoreMemory  DataStoreName=MaterialID  InitialValue=Elements(id).Material(1).ID  OutDataType=sfix(16)  OutScaling=2^0
  Data Store Read : DataStoreRead  DataStoreName=Node1ID  SampleTime=SampleRate
  Data Store Read10 : DataStoreRead  DataStoreName=MaterialE  SampleTime=SampleRate
  Data Store Read11 : DataStoreRead  DataStoreName=Area  SampleTime=SampleRate
  Data Store Read12 : DataStoreRead  DataStoreName=Inertia  SampleTime=SampleRate
  Data Store Read2 : DataStoreRead  DataStoreName=Node1Xcoord  SampleTime=SampleRate
  Data Store Read3 : DataStoreRead  DataStoreName=Node1Ycoord  SampleTime=SampleRate
  Data Store Read5 : DataStoreRead  DataStoreName=Node2ID  SampleTime=SampleRate
  Data Store Read6 : DataStoreRead  DataStoreName=Node2Xcoord  SampleTime=SampleRate
  Data Store Read7 : DataStoreRead  DataStoreName=Node2Ycoord  SampleTime=SampleRate
  Element : Outport  OutDataType=sfix(16)  OutScaling=2^0
  wires:
  Bus Creator/1 -> Element/1
  Data Store Read/1 -> Bus Creator/1  "Node1 ID"
  Data Store Read2/1 -> Bus Creator/2  "Node1 Xcoord"
  Data Store Read3/1 -> Bus Creator/3  "Node1 Ycoord"
  Data Store Read5/1 -> Bus Creator/4  "Node2 ID"
  Data Store Read6/1 -> Bus Creator/5  "Node2 Xcoord"
  Data Store Read7/1 -> Bus Creator/6  "Node2 Ycoord"
  Data Store Read10/1 -> Bus Creator/7  "Material E"
  Data Store Read11/1 -> Bus Creator/8  "Area"
  Data Store Read12/1 -> Bus Creator/9  "Inertia"

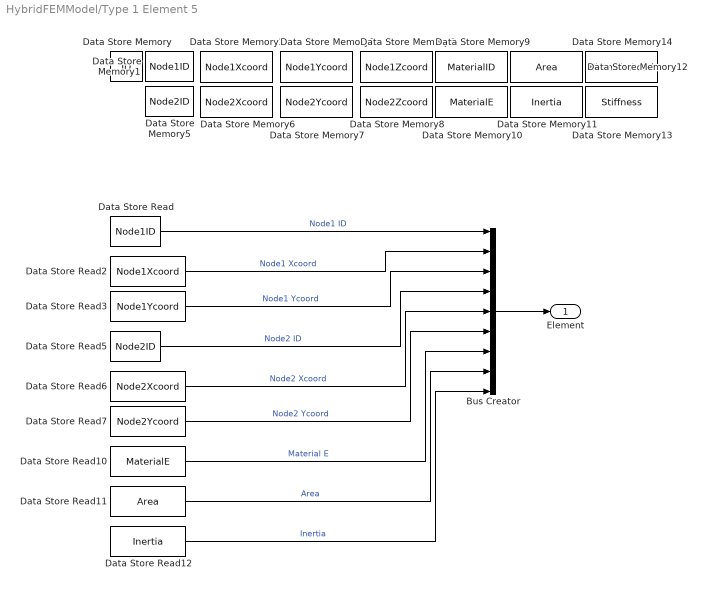
== system HybridFEMModel/Type 1 Element 5 ==
  Bus Creator : BusCreator  Inputs=9
  Data Store Memory : DataStoreMemory  DataStoreName=ID  InitialValue=Elements(id).ID  OutDataType=sfix(16)  OutScaling=2^0
  Data Store Memory1 : DataStoreMemory  DataStoreName=Node1ID  InitialValue=Elements(id).Nodes(1).ID  OutDataType=sfix(16)  OutScaling=2^0
  Data Store Memory10 : DataStoreMemory  DataStoreName=MaterialE  InitialValue=Elements(id).Material(1).E  OutDataType=sfix(16)  OutScaling=2^0
  Data Store Memory11 : DataStoreMemory  DataStoreName=Inertia  InitialValue=Elements(id).Inertia  OutDataType=sfix(16)  OutScaling=2^0
  Data Store Memory12 : DataStoreMemory  DataStoreName=Area  InitialValue=Elements(id).Area  OutDataType=sfix(16)  OutScaling=2^0
  Data Store Memory13 : DataStoreMemory  DataStoreName=Stiffness  InitialValue=Elements(id).Stiffness  OutDataType=sfix(16)  OutScaling=2^0
  Data Store Memory14 : DataStoreMemory  DataStoreName=ElemDistLoad  InitialValue=Elements(id).ElemDistLoad  OutDataType=sfix(16)  OutScaling=2^0
  Data Store Memory2 : DataStoreMemory  DataStoreName=Node1Xcoord  InitialValue=Elements(id).Nodes(1).Xcoord  OutDataType=sfix(16)  OutScaling=2^0
  Data Store Memory3 : DataStoreMemory  DataStoreName=Node1Ycoord  InitialValue=Elements(id).Nodes(1).Ycoord  OutDataType=sfix(16)  OutScaling=2^0
  Data Store Memory4 : DataStoreMemory  DataStoreName=Node1Zcoord  InitialValue=Elements(id).Nodes(1).Zcoord  OutDataType=sfix(16)  OutScaling=2^0
  Data Store Memory5 : DataStoreMemory  DataStoreName=Node2ID  InitialValue=Elements(id).Nodes(2).ID  OutDataType=sfix(16)  OutScaling=2^0
  Data Store Memory6 : DataStoreMemory  DataStoreName=Node2Xcoord  InitialValue=Elements(id).Nodes(2).Xcoord  OutDataType=sfix(16)  OutScaling=2^0
  Data Store Memory7 : DataStoreMemory  DataStoreName=Node2Ycoord  InitialValue=Elements(id).Nodes(2).Ycoord  OutDataType=sfix(16)  OutScaling=2^0
  Data Store Memory8 : DataStoreMemory  DataStoreName=Node2Zcoord  InitialValue=Elements(id).Nodes(2).Zcoord  OutDataType=sfix(16)  OutScaling=2^0
  Data Store Memory9 : DataStoreMemory  DataStoreName=MaterialID  InitialValue=Elements(id).Material(1).ID  OutDataType=sfix(16)  OutScaling=2^0
  Data Store Read : DataStoreRead  DataStoreName=Node1ID  SampleTime=SampleRate
  Data Store Read10 : DataStoreRead  DataStoreName=MaterialE  SampleTime=SampleRate
  Data Store Read11 : DataStoreRead  DataStoreName=Area  SampleTime=SampleRate
  Data Store Read12 : DataStoreRead  DataStoreName=Inertia  SampleTime=SampleRate
  Data Store Read2 : DataStoreRead  DataStoreName=Node1Xcoord  SampleTime=SampleRate
  Data Store Read3 : DataStoreRead  DataStoreName=Node1Ycoord  SampleTime=SampleRate
  Data Store Read5 : DataStoreRead  DataStoreName=Node2ID  SampleTime=SampleRate
  Data Store Read6 : DataStoreRead  DataStoreName=Node2Xcoord  SampleTime=SampleRate
  Data Store Read7 : DataStoreRead  DataStoreName=Node2Ycoord  SampleTime=SampleRate
  Element : Outport  OutDataType=sfix(16)  OutScaling=2^0
  wires:
  Data Store Read12/1 -> Bus Creator/9  "Inertia"
  Data Store Read11/1 -> Bus Creator/8  "Area"
  Data Store Read10/1 -> Bus Creator/7  "Material E"
  Data Store Read7/1 -> Bus Creator/6  "Node2 Ycoord"
  Data Store Read6/1 -> Bus Creator/5  "Node2 Xcoord"
  Data Store Read5/1 -> Bus Creator/4  "Node2 ID"
  Data Store Read3/1 -> Bus Creator/3  "Node1 Ycoord"
  Data Store Read2/1 -> Bus Creator/2  "Node1 Xcoord"
  Data Store Read/1 -> Bus Creator/1  "Node1 ID"
  Bus Creator/1 -> Element/1

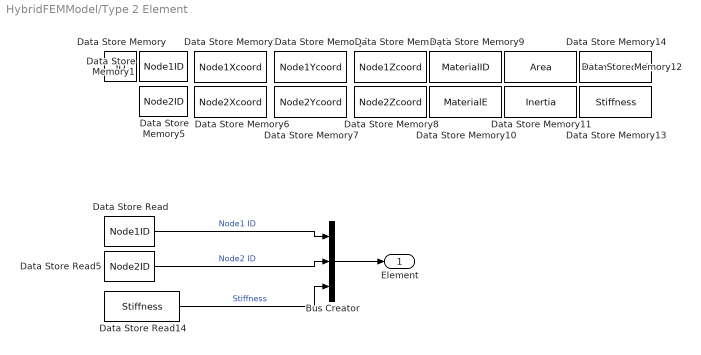
== system HybridFEMModel/Type 2 Element ==
  Bus Creator : BusCreator  Inputs=3
  Data Store Memory : DataStoreMemory  DataStoreName=ID  InitialValue=Elements(id).ID  OutDataType=sfix(16)  OutScaling=2^0
  Data Store Memory1 : DataStoreMemory  DataStoreName=Node1ID  InitialValue=Elements(id).Nodes(1).ID  OutDataType=sfix(16)  OutScaling=2^0
  Data Store Memory10 : DataStoreMemory  DataStoreName=MaterialE  InitialValue=Elements(id).Material(1).E  OutDataType=sfix(16)  OutScaling=2^0
  Data Store Memory11 : DataStoreMemory  DataStoreName=Inertia  InitialValue=Elements(id).Inertia  OutDataType=sfix(16)  OutScaling=2^0
  Data Store Memory12 : DataStoreMemory  DataStoreName=Area  InitialValue=Elements(id).Area  OutDataType=sfix(16)  OutScaling=2^0
  Data Store Memory13 : DataStoreMemory  DataStoreName=Stiffness  InitialValue=Elements(id).Stiffness  OutDataType=sfix(16)  OutScaling=2^0
  Data Store Memory14 : DataStoreMemory  DataStoreName=ElemDistLoad  InitialValue=Elements(id).ElemDistLoad  OutDataType=sfix(16)  OutScaling=2^0
  Data Store Memory2 : DataStoreMemory  DataStoreName=Node1Xcoord  InitialValue=Elements(id).Nodes(1).Xcoord  OutDataType=sfix(16)  OutScaling=2^0
  Data Store Memory3 : DataStoreMemory  DataStoreName=Node1Ycoord  InitialValue=Elements(id).Nodes(1).Ycoord  OutDataType=sfix(16)  OutScaling=2^0
  Data Store Memory4 : DataStoreMemory  DataStoreName=Node1Zcoord  InitialValue=Elements(id).Nodes(1).Zcoord  OutDataType=sfix(16)  OutScaling=2^0
  Data Store Memory5 : DataStoreMemory  DataStoreName=Node2ID  InitialValue=Elements(id).Nodes(2).ID  OutDataType=sfix(16)  OutScaling=2^0
  Data Store Memory6 : DataStoreMemory  DataStoreName=Node2Xcoord  InitialValue=Elements(id).Nodes(2).Xcoord  OutDataType=sfix(16)  OutScaling=2^0
  Data Store Memory7 : DataStoreMemory  DataStoreName=Node2Ycoord  InitialValue=Elements(id).Nodes(2).Ycoord  OutDataType=sfix(16)  OutScaling=2^0
  Data Store Memory8 : DataStoreMemory  DataStoreName=Node2Zcoord  InitialValue=Elements(id).Nodes(2).Zcoord  OutDataType=sfix(16)  OutScaling=2^0
  Data Store Memory9 : DataStoreMemory  DataStoreName=MaterialID  InitialValue=Elements(id).Material(1).ID  OutDataType=sfix(16)  OutScaling=2^0
  Data Store Read : DataStoreRead  DataStoreName=Node1ID  SampleTime=SampleRate
  Data Store Read14 : DataStoreRead  DataStoreName=Stiffness  SampleTime=SampleRate
  Data Store Read5 : DataStoreRead  DataStoreName=Node2ID  SampleTime=SampleRate
  Element : Outport  OutDataType=sfix(16)  OutScaling=2^0
  wires:
  Data Store Read14/1 -> Bus Creator/3  "Stiffness"
  Data Store Read5/1 -> Bus Creator/2  "Node2 ID"
  Data Store Read/1 -> Bus Creator/1  "Node1 ID"
  Bus Creator/1 -> Element/1

== system HybridFEMModel/Generate Acceleration Vector/Step Count ==
  Increment Stored Integer : simulink/Additional Math & Discrete/Additional Math: Increment - Decrement/Increment Stored Integer  SystemSampleTime=-1
  step count : simulink/Sources/Counter Free-Running  SystemSampleTime=-1  NumBits=32  tsamp=SampleRate
  Step Count : Outport  OutDataType=sfix(16)  OutScaling=2^0
  wires:
  step count/1 -> Increment Stored Integer/1
  Increment Stored Integer/1 -> Step Count/1

== matlab function Generate Type 2 Element Restoring Force/Type 2 Element RF ==
  data: Nodes output inherited; Element input inherited; RF output inherited; NumFreeDOF input inherited; Displacement input inherited
% get restoring force for the element
% returns (6x1) restoring force vector of element in global coordinates
function [Nodes,RF] = fcn(Element, NumFreeDOF, Displacement)

%% Input mapping
Node1ID = Element(1);
Node2ID = Element(2);
Stiffness = Element(3);
Nodes = [Node1ID,Node2ID];

% Get distance between nodes
I1 = Node1ID;
I2 = Node2ID;

% preset arrays
SE = zeros(6,6);
    
SE(1, 1) = Stiffness;
SE(1, 4) = -Stiffness;
SE(4, 4) = Stiffness;
SE(4, 1) = SE(1,4);
%create the displacement Ue (6x1) vector of the element in global coordinates
Ue = zeros(6, 1);
if (I1 * 3) <= NumFreeDOF
    Ue(1, 1) = Displacement(I1 * 3 - 2, 1);
    Ue(2, 1) = Displacement(I1 * 3 - 1, 1);
    Ue(3, 1) = Displacement(I1 * 3, 1);
end
if (I2 * 3) <= NumFreeDOF
    Ue(4, 1) = Displacement(I2 * 3 - 2, 1);
    Ue(5, 1) = Displacement(I2 * 3 - 1, 1);
    Ue(6, 1) = Displacement(I2 * 3, 1);
end
RF = SE*Ue;  %resisting (6x1) resisting force vector of element in global coordinates
